simulink model "testStateFeedback1"  (R2019b)
settings: Solver=VariableStepAuto  StartTime=0.0  StopTime=10.0  RelTol=1e-3
values from neighbouring files (symbols this model uses):
  Ax = [0 1 0 0; 0 0 obj.g 0; 0 0 0 1; 0 0 0 0]    [SubSysController.m]    (also in linearizationB.m = double(subs(Ax,g,9.81)))
  Bx = [0; 0; 0; 1/obj.Iyy]    [SubSysController.m]    (also in linearizationB.m = double(subs(Bx,Iyy,1.657171e-5)))
  K = 1    [AdmittanceCtrlComplete.m]    (also in linearizationB.m = place(Ax,Bx,p); numerical_derivatives.m)
settings Model: Creator=toto  LastModifiedBy=toto

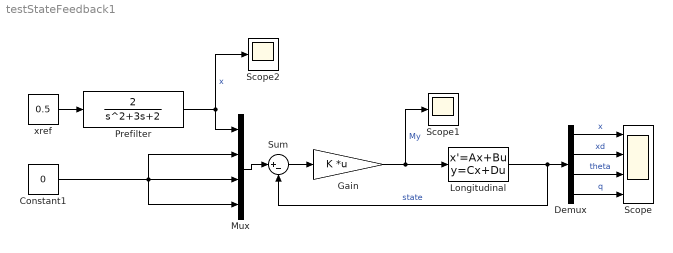
== system testStateFeedback1 ==
  Constant1 : Constant  Value=0
  Demux : Demux
  Gain : Gain  Gain=K  Multiplication=Matrix(K*u) (u vector)
  Longitudinal : StateSpace  A=Ax  B=Bx  C=eye(4)  D=zeros(4,1)  InitialCondition=0
  Mux : Mux
  Prefilter : TransferFcn  Numerator=[2]  Denominator=[1 3 2]
  Scope : Scope  NumInputPorts=4
  Scope1 : Scope
  Scope2 : Scope
  Sum : Sum  Inputs=|+-
  xref : Constant  Value=0.5
  wires:
  Sum/1 -> Gain/1
  Gain/1 -> Scope1/1, Longitudinal/1  "My"
  Longitudinal/1 -> Demux/1, Sum/2  "state"
  Demux/1 -> Scope/1  "x"
  Demux/2 -> Scope/2  "xd"
  Demux/3 -> Scope/3  "theta"
  Demux/4 -> Scope/4  "q"
  xref/1 -> Prefilter/1
  Prefilter/1 -> Mux/1, Scope2/1  "x"
  Mux/1 -> Sum/1
  Constant1/1 -> Mux/2, Mux/3, Mux/4
